simulink model "SILTest"  (R2018b)
settings: Solver=FixedStepDiscrete  StartTime=0.0  StopTime=10.0  FixedStep=SimStep  RelTol=1e-3
values from neighbouring files (symbols this model uses):
  SimStep = 0.1    [init.m]
  Tbl = createCfsTbl(TblVals, 'Tbl', 'ValidateTbl')    [init.m]
libraries: cfs_library x6, simulink x5
settings Model: Creator=slentine  LastModifiedBy=slentine
settings OptimizationCC: DefaultParameterBehavior=Inlined  EnhancedBackFolding=on  PassReuseOutputArgsAs=Individual arguments  OptimizeBlockOrder=speed  DifferentSizesBufferReuse=on  OptimizationCustomize=off
settings DebuggingCC: ParameterTunabilityLossMsg=error
settings SFSimCC: MATLABDynamicMemAlloc=off
settings RTWCC: SystemTargetFile=cfs_ert.tlc  GenCodeOnly=on  TemplateMakefile=ert_default_tmf  Description=NASA CFS Target File  GenerateReport=on  IncludeHyperlinkInReport=on  LaunchReport=on  GenerateTraceInfo=on  GenerateTraceReport=on  GenerateTraceReportSl=on  GenerateTraceReportSf=on  GenerateTraceReportEml=on
settings CodeAppCC: ForceParamTrailComments=on  IgnoreCustomStorageClasses=off  OperatorAnnotations=on  SimulinkDataObjDesc=on  SFDataObjDesc=on  InsertBlockDesc=on
settings STFCustomTargetCC: TargetLangStandard=C99 (ISO)  MultiwordLength=256  CombineOutputUpdateFcns=on  ERTCustomFileBanners=on  SupportContinuousTime=off  SupportNonInlinedSFcns=off  RemoveResetFunc=on  MATLABClassNameForMDSCustomization=Simulink.SoftwareTarget.ERTCustomization  UseToolchainInfoCompliant=on  SystemTargetFile=cfs_ert.tlc
settings ERTTargetCC: TargetLangStandard=C99 (ISO)  ParMdlRefBuildCompliant=off  CompOptLevelCompliant=off  ConcurrentExecutionCompliant=off  ModelStepFunctionPrototypeControlCompliant=off  CPPClassGenCompliant=off  InlinedParameterPlacement=NonHierarchical  ERTCustomFileTemplate=cfs_interface.tlc

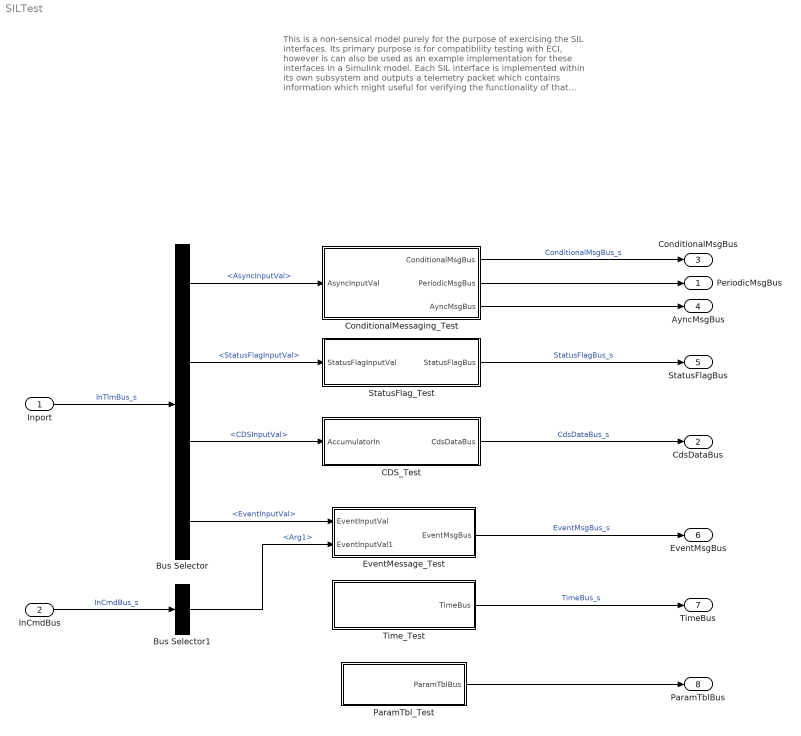
== system SILTest ==
  note: This is a non-sensical model purely for the purpose of exercising
      | the SIL interfaces. Its primary purpose is for compatibility testing
      | with ECI, however is can also be used as an example implementation
      | for these interfaces in a Simulink model.
      |
      | Each SIL interface is implemented within its own subsystem and
      | outputs a telemetry packet which contains information which might
      | useful for verifying the functionality of that particular feature. The
      | verification is not performed automatically at this time.
      |
      | Note that the packet ingest and packet output functionality are tested
      | implicitly in the inputs and outputs used for/generated by the other
      | features.
  Inport : Inport  OutDataTypeStr=Bus: InTlmBus  Interpolate=off  BusOutputAsStruct=on
  InCmdBus : Inport  Port=2  OutDataTypeStr=Bus: InCmdBus  Interpolate=off  BusOutputAsStruct=on
  Bus Selector : BusSelector  OutputSignals=AsyncInputVal,StatusFlagInputVal,CDSInputVal,EventInputVal
  Bus Selector1 : BusSelector  OutputSignals=Arg1
  CDS_Test : Subsystem
  ConditionalMessaging_Test : Subsystem
  EventMessage_Test : Subsystem
  ParamTbl_Test : Subsystem
  StatusFlag_Test : Subsystem
  Time_Test : Subsystem
  PeriodicMsgBus : Outport  OutDataTypeStr=Bus: PeriodicMsgBus
  CdsDataBus : Outport  Port=2  OutDataTypeStr=Bus: CdsDataBus
  ConditionalMsgBus : Outport  Port=3  OutDataTypeStr=Bus: ConditionalMsgBus
  AyncMsgBus : Outport  Port=4  OutDataTypeStr=Bus: AyncMsgBus
  StatusFlagBus : Outport  Port=5  OutDataTypeStr=Bus: StatusFlagBus
  EventMsgBus : Outport  Port=6  OutDataTypeStr=Bus: EventMsgBus
  TimeBus : Outport  Port=7  OutDataTypeStr=Bus: TimeBus
  ParamTblBus : Outport  Port=8  OutDataTypeStr=Bus: ParamTblBus
  wires:
  Inport/1 -> Bus Selector/1  "InTlmBus_s"
  CDS_Test/1(CdsDataBus) -> CdsDataBus/1  "CdsDataBus_s"
  ConditionalMessaging_Test/2(PeriodicMsgBus) -> PeriodicMsgBus/1
  ConditionalMessaging_Test/1(ConditionalMsgBus) -> ConditionalMsgBus/1  "ConditionalMsgBus_s"
  ConditionalMessaging_Test/3(AyncMsgBus) -> AyncMsgBus/1
  Bus Selector/1 -> ConditionalMessaging_Test/1(AsyncInputVal)  "<AsyncInputVal>"
  StatusFlag_Test/1(StatusFlagBus) -> StatusFlagBus/1  "StatusFlagBus_s"
  Bus Selector/3 -> CDS_Test/1(AccumulatorIn)  "<CDSInputVal>"
  Bus Selector/2 -> StatusFlag_Test/1(StatusFlagInputVal)  "<StatusFlagInputVal>"
  Bus Selector/4 -> EventMessage_Test/1(EventInputVal)  "<EventInputVal>"
  EventMessage_Test/1(EventMsgBus) -> EventMsgBus/1  "EventMsgBus_s"
  Time_Test/1(TimeBus) -> TimeBus/1  "TimeBus_s"
  ParamTbl_Test/1(ParamTblBus) -> ParamTblBus/1
  InCmdBus/1 -> Bus Selector1/1  "InCmdBus_s"
  Bus Selector1/1 -> EventMessage_Test/2(EventInputVal1)  "<Arg1>"

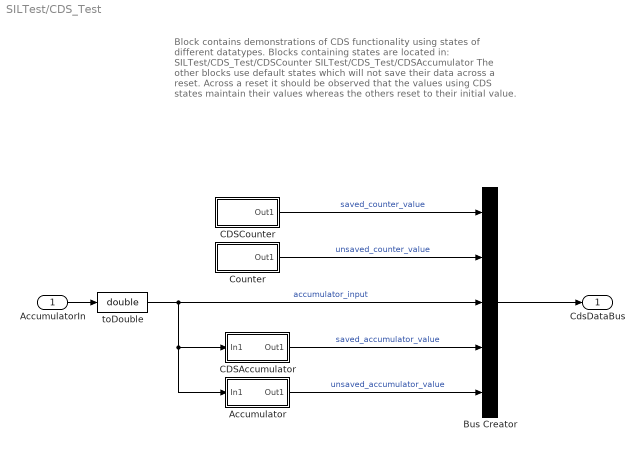
== system SILTest/CDS_Test ==
  note: Block contains demonstrations of CDS functionality using states
      | of different datatypes. Blocks containing states are located in:
      |
      | SILTest/CDS_Test/CDSCounter
      | SILTest/CDS_Test/CDSAccumulator
      |
      | The other blocks use default states which will not save their data
      | across a reset.
      |
      | Across a reset it should be observed that the values using CDS states
      | maintain their values whereas the others reset to their initial value.
  AccumulatorIn : Inport
  Accumulator : Subsystem
  Bus Creator : BusCreator  Inputs=5  OutDataTypeStr=Bus: CdsDataBus  NonVirtualBus=on
  CDSAccumulator : Subsystem
  CDSCounter : Subsystem
  Counter : Subsystem
  toDouble : DataTypeConversion  OutDataTypeStr=double
  CdsDataBus : Outport  OutDataTypeStr=Bus: CdsDataBus
  wires:
  Bus Creator/1 -> CdsDataBus/1
  Counter/1(Out1) -> Bus Creator/2  "unsaved_counter_value"
  AccumulatorIn/1 -> toDouble/1
  CDSAccumulator/1(Out1) -> Bus Creator/4  "saved_accumulator_value"
  toDouble/1 -> Accumulator/1(In1), CDSAccumulator/1(In1), Bus Creator/3  "accumulator_input"
  CDSCounter/1(Out1) -> Bus Creator/1  "saved_counter_value"
  Accumulator/1(Out1) -> Bus Creator/5  "unsaved_accumulator_value"

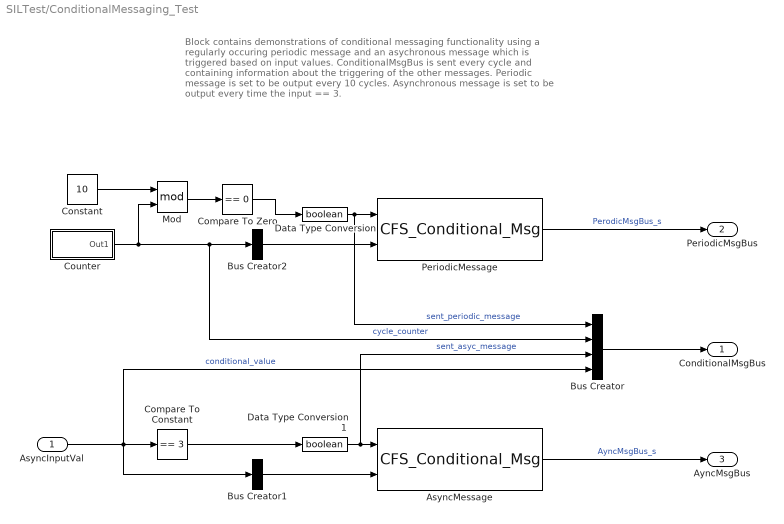
== system SILTest/ConditionalMessaging_Test ==
  note: Block contains demonstrations of conditional messaging functionality using
      | a regularly occuring periodic message and an asychronous message which
      | is triggered based on input values. ConditionalMsgBus is sent every cycle
      | and containing information about the triggering of the other messages.
      |
      | Periodic message is set to be output every 10 cycles.
      |
      | Asynchronous message is set to be output every time the input == 3.
  AsyncInputVal : Inport  OutDataTypeStr=uint8
  AsyncMessage : cfs_library/CFS_Conditional_Msg  bus_name=[]  bus_type=Bus: AyncMsgBus  block_sid=[]
      settings: SourceProductName=CFS Blockset
  Bus Creator : BusCreator  Inputs=4  OutDataTypeStr=Bus: ConditionalMsgBus  NonVirtualBus=on
  Bus Creator1 : BusCreator  Inputs=1  OutDataTypeStr=Bus: AyncMsgBus  NonVirtualBus=on
  Bus Creator2 : BusCreator  Inputs=1  OutDataTypeStr=Bus: PeriodicMsgBus  NonVirtualBus=on
  Compare To Constant : simulink/Logic and Bit Operations/Compare To Constant  relop===  const=3  OutDataTypeStr=boolean
  Compare To Zero : simulink/Logic and Bit Operations/Compare To Zero  relop===  OutDataTypeStr=boolean
  Constant : Constant  Value=10  OutDataTypeStr=uint8
  Counter : Subsystem
  Data Type Conversion : DataTypeConversion  OutDataTypeStr=boolean
  Data Type Conversion1 : DataTypeConversion  OutDataTypeStr=boolean
  Mod : Math  Operator=mod  SaturateOnIntegerOverflow=on
  PeriodicMessage : cfs_library/CFS_Conditional_Msg  bus_name=[]  bus_type=Bus: PeriodicMsgBus  block_sid=[]
      settings: SourceProductName=CFS Blockset
  ConditionalMsgBus : Outport
  PeriodicMsgBus : Outport  Port=2
  AyncMsgBus : Outport  Port=3
  wires:
  Data Type Conversion/1 -> Bus Creator/1, PeriodicMessage/1  "sent_periodic_message"
  PeriodicMessage/1 -> PeriodicMsgBus/1  "PerodicMsgBus_s"
  Bus Creator/1 -> ConditionalMsgBus/1
  Data Type Conversion1/1 -> Bus Creator/3, AsyncMessage/1  "sent_asyc_message"
  Bus Creator1/1 -> AsyncMessage/2
  AsyncMessage/1 -> AyncMsgBus/1  "AyncMsgBus_s"
  Bus Creator2/1 -> PeriodicMessage/2
  Counter/1(Out1) -> Mod/2, Bus Creator/2, Bus Creator2/1  "cycle_counter"
  Mod/1 -> Compare To Zero/1
  Constant/1 -> Mod/1
  Compare To Zero/1 -> Data Type Conversion/1
  Compare To Constant/1 -> Data Type Conversion1/1
  AsyncInputVal/1 -> Bus Creator/4, Bus Creator1/1, Compare To Constant/1  "conditional_value"

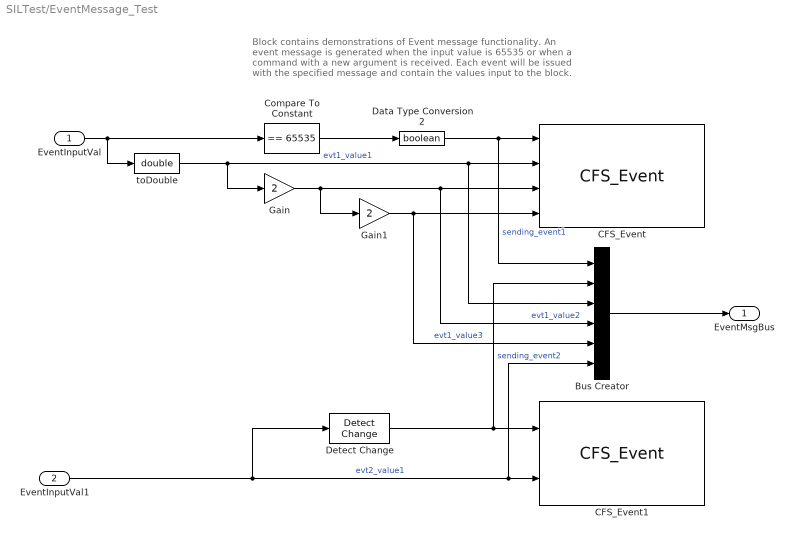
== system SILTest/EventMessage_Test ==
  note: Block contains demonstrations of Event message functionality.
      |
      | An event message is generated when the input value is 65535
      | or when a command with a new argument is received. Each event
      | will be issued with the specified message and contain the values
      | input to the block.
  EventInputVal : Inport
  EventInputVal1 : Inport  Port=2
  Bus Creator : BusCreator  Inputs=6  OutDataTypeStr=Bus: EventMsgBus  NonVirtualBus=on
  CFS_Event : cfs_library/CFS_Event  event_id=Event1_ID  event_type=Event1_Type  event_mask=Event1_Mask  string_data=Event1_Message  fmt_string=uint8(['Loc: %s, Value: %f, Value*2: %f, Value*4: %f' 0])  num_data_ports=Event1_DataPorts  block_sid=0
      settings: SourceProductName=CFS Blockset
  CFS_Event1 : cfs_library/CFS_Event  event_id=Event2_ID  event_type=Event2_Type  event_mask=Event2_Mask  string_data=Event2_Message  fmt_string=uint8(['Loc: %s, Command argument value: %f' 0])  num_data_ports=Event2_DataPorts  block_sid=0
      settings: SourceProductName=CFS Blockset
  Compare To Constant : simulink/Logic and Bit Operations/Compare To Constant  relop===  const=65535  OutDataTypeStr=boolean
  Data Type Conversion2 : DataTypeConversion  OutDataTypeStr=boolean
  Detect Change : simulink/Logic and Bit Operations/Detect Change  vinit=0  OutDataTypeStr=boolean
  Gain : Gain  Gain=2
  Gain1 : Gain  Gain=2
  toDouble : DataTypeConversion  OutDataTypeStr=double
  EventMsgBus : Outport
  wires:
  Gain1/1 -> Bus Creator/5, CFS_Event/4  "evt1_value3"
  Data Type Conversion2/1 -> CFS_Event/1, Bus Creator/1  "sending_event1"
  Compare To Constant/1 -> Data Type Conversion2/1
  Bus Creator/1 -> EventMsgBus/1
  EventInputVal/1 -> Compare To Constant/1, toDouble/1
  toDouble/1 -> Gain/1, Bus Creator/3, CFS_Event/2  "evt1_value1"
  Gain/1 -> Gain1/1, Bus Creator/4, CFS_Event/3  "evt1_value2"
  EventInputVal1/1 -> Detect Change/1, Bus Creator/6, CFS_Event1/2  "evt2_value1"
  Detect Change/1 -> Bus Creator/2, CFS_Event1/1  "sending_event2"

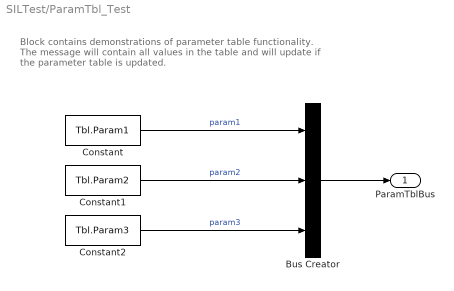
== system SILTest/ParamTbl_Test ==
  note: Block contains demonstrations of parameter table functionality.
      |
      | The message will contain all values in the table and will update
      | if the parameter table is updated.
  Bus Creator : BusCreator  Inputs=3  OutDataTypeStr=Bus: ParamTblBus  NonVirtualBus=on
  Constant : Constant  Value=Tbl.Param1
  Constant1 : Constant  Value=Tbl.Param2
  Constant2 : Constant  Value=Tbl.Param3
  ParamTblBus : Outport  OutDataTypeStr=Bus: ParamTblBus
  wires:
  Constant/1 -> Bus Creator/1  "param1"
  Bus Creator/1 -> ParamTblBus/1
  Constant1/1 -> Bus Creator/2  "param2"
  Constant2/1 -> Bus Creator/3  "param3"

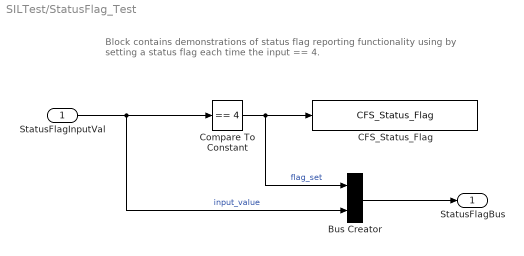
== system SILTest/StatusFlag_Test ==
  note: Block contains demonstrations of status flag reporting functionality using
      | by setting a status flag each time the input == 4.
  StatusFlagInputVal : Inport  OutDataTypeStr=uint8
  Bus Creator : BusCreator  Inputs=2  OutDataTypeStr=Bus: StatusFlagBus  NonVirtualBus=on
  CFS_Status_Flag : cfs_library/CFS_Status_Flag  fdc_id=Flag_ID  block_sid=0
      settings: SourceProductName=CFS Blockset
  Compare To Constant : simulink/Logic and Bit Operations/Compare To Constant  relop===  const=4  OutDataTypeStr=boolean
  StatusFlagBus : Outport
  wires:
  Compare To Constant/1 -> Bus Creator/1, CFS_Status_Flag/1  "flag_set"
  Bus Creator/1 -> StatusFlagBus/1
  StatusFlagInputVal/1 -> Bus Creator/2, Compare To Constant/1  "input_value"

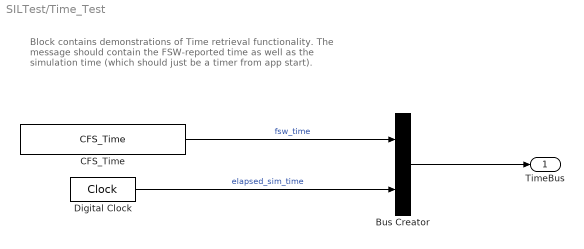
== system SILTest/Time_Test ==
  note: Block contains demonstrations of Time retrieval functionality.
      |
      | The message should contain the FSW-reported time as well as
      | the simulation time (which should just be a timer from app start).
  Bus Creator : BusCreator  Inputs=2  OutDataTypeStr=Bus: TimeBus  NonVirtualBus=on
  CFS_Time : cfs_library/CFS_Time  SFunctionSpec=double y1 = get_gps(double p1)  SParameter1=Time_epoch  SParameter2=0.1
      settings: SourceProductName=CFS Blockset
  Digital Clock : DigitalClock  SampleTime=SimStep
  TimeBus : Outport
  wires:
  Bus Creator/1 -> TimeBus/1
  CFS_Time/1 -> Bus Creator/1  "fsw_time"
  Digital Clock/1 -> Bus Creator/2  "elapsed_sim_time"

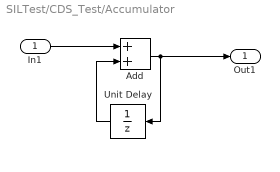
== system SILTest/CDS_Test/Accumulator ==
  In1 : Inport
  Add : Sum
  Unit Delay : UnitDelay  SampleTime=-1
  Out1 : Outport
  wires:
  Unit Delay/1 -> Add/2
  Add/1 -> Unit Delay/1, Out1/1
  In1/1 -> Add/1

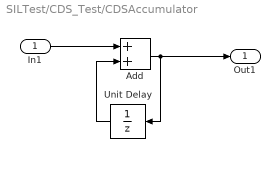
== system SILTest/CDS_Test/CDSAccumulator ==
  In1 : Inport
  Add : Sum
  Unit Delay : UnitDelay  SampleTime=-1  StateName=double_accumulator_state  StateMustResolveToSignalObject=on
  Out1 : Outport
  wires:
  In1/1 -> Add/1
  Add/1 -> Out1/1, Unit Delay/1
  Unit Delay/1 -> Add/2

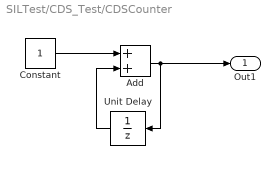
== system SILTest/CDS_Test/CDSCounter ==
  Add : Sum
  Constant : Constant  OutDataTypeStr=uint8
  Unit Delay : UnitDelay  SampleTime=-1  StateName=uint8_counter_state  StateMustResolveToSignalObject=on
  Out1 : Outport
  wires:
  Unit Delay/1 -> Add/2
  Add/1 -> Unit Delay/1, Out1/1
  Constant/1 -> Add/1

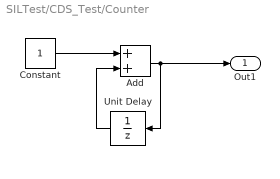
== system SILTest/CDS_Test/Counter ==
  Add : Sum
  Constant : Constant  OutDataTypeStr=uint8
  Unit Delay : UnitDelay  SampleTime=-1
  Out1 : Outport
  wires:
  Constant/1 -> Add/1
  Add/1 -> Out1/1, Unit Delay/1
  Unit Delay/1 -> Add/2

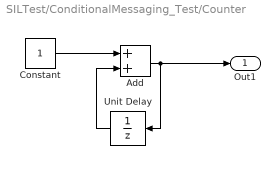
== system SILTest/ConditionalMessaging_Test/Counter ==
  Add : Sum
  Constant : Constant  OutDataTypeStr=uint8
  Unit Delay : UnitDelay  SampleTime=-1
  Out1 : Outport
  wires:
  Constant/1 -> Add/1
  Add/1 -> Out1/1, Unit Delay/1
  Unit Delay/1 -> Add/2
